simulink subsystem "EV_ThorneFleissner"  (R2020b)
settings: Solver=VariableStepAuto  StartTime=0.0  StopTime=10.0  RelTol=1e-3
values from neighbouring files (symbols this model uses):
  Map = im2double(Map).*255    [Configuration.m]    (also in ConfigurationCreation.m)
undefined symbols (not defined in the file or in its folder): initX
libraries: simulink_extras x6, dspnetwork x3, pid_lib x2, simulink x2
(part 2 of 2)

== matlab function EV_ThorneFleissner/Sensor Input Block/left circle check ==
  data: map input; rli output; x input; y input; r input
function rli = circle(map,x,y,r)
%x and y are the coordinates of the center of the circle
%r is the radius of the circle
region = map(y-r:y+r, x-r:x+r); %matlab indexes the opposite of images, select s square around the circle 
[MX,MY] = meshgrid(-r:r, -r:r);
mask = MX.^2 + MY.^2 <= r^2;
rli = sum(sum(region.*double(mask))) / sum(sum(mask));%sum(sum(mask));
rli = round(rli * .7 + 10);
end

== matlab function EV_ThorneFleissner/Sensor Input Block/right circle check ==
  data: map input; rli output; x input; y input; r input
function rli = circle(map,x,y,r)
%x and y are the coordinates of the center of the circle
%r is the radius of the circle
region = map(y-r:y+r, x-r:x+r); %matlab indexes the opposite of images, select s square around the circle 
[MX,MY] = meshgrid(-r:r, -r:r);
mask = MX.^2 + MY.^2 <= r^2;
rli = sum(sum(region.*double(mask))) / sum(sum(mask));%sum(sum(mask));
rli = round(rli*.7 + 10);
end
